simulink model "oneThrCtrl_th"  (R2018b)
settings: Solver=VariableStepAuto  StartTime=0.0  StopTime=10.0  RelTol=1e-3
values from neighbouring files (symbols this model uses):
  alti_sp = 0    [oneThrCtrl_ts.m]
  eulerAng = [0;0;0]*pi/180    [oneThrCtrl_ts.m]
  flow = [0;0;0]    [oneThrCtrl_ts.m]
  OwB = [0;0;0]    [oneThrCtrl_ts.m]
  pitch_sp = 0*pi/180    (= 0)    [oneThrCtrl_ts.m]
  Rcm_o = [0;0;0]    [oneThrCtrl_ts.m]
  roll_sp = 0*pi/180    (= 0)    [oneThrCtrl_ts.m]
  Vcm_o = zeros(3,1)    [oneThrCtrl_ts.m]
  yaw_sp = 5*pi/180    (= 0.0872664625997)    [oneThrCtrl_ts.m]
libraries: oneTetCtrllr_cl x1
settings Model: Creator=asiddiq2  LastModifiedBy=asiddiq2

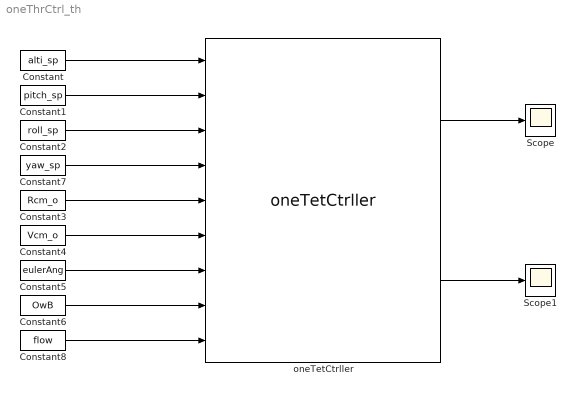
== system oneThrCtrl_th ==
  Constant : Constant  Value=alti_sp  VectorParams1D=off
  Constant1 : Constant  Value=pitch_sp  VectorParams1D=off
  Constant2 : Constant  Value=roll_sp  VectorParams1D=off
  Constant3 : Constant  Value=Rcm_o  VectorParams1D=off
  Constant4 : Constant  Value=Vcm_o  VectorParams1D=off
  Constant5 : Constant  Value=eulerAng  VectorParams1D=off
  Constant6 : Constant  Value=OwB  VectorParams1D=off
  Constant7 : Constant  Value=yaw_sp  VectorParams1D=off
  Constant8 : Constant  Value=flow  VectorParams1D=off
  Scope : Scope
  Scope1 : Scope
  oneTetCtrller : oneTetCtrllr_cl/oneTetCtrller  SystemSampleTime=-1
  wires:
  Constant1/1 -> oneTetCtrller/2
  Constant8/1 -> oneTetCtrller/9
  Constant4/1 -> oneTetCtrller/6
  Constant7/1 -> oneTetCtrller/4
  Constant6/1 -> oneTetCtrller/8
  Constant5/1 -> oneTetCtrller/7
  Constant3/1 -> oneTetCtrller/5
  Constant2/1 -> oneTetCtrller/3
  Constant/1 -> oneTetCtrller/1
  oneTetCtrller/2 -> Scope1/1
  oneTetCtrller/1 -> Scope/1
